simulink model "utolso"  (R2023b)
settings: Solver=FixedStepAuto  StartTime=0.0  StopTime=100  FixedStep=0.01  RelTol=1e-3
values from neighbouring files (symbols this model uses):
  A = [2 5 2.3; 1 0 3; 0 -4.1 5]    [elso_ora.m]    (also in laborXI.m = [0 1;-k/m -b/m])
  Ah = [A B; 0 0 0]    [laborXI.m]
  B = [1;-1;-2]    [elso_ora.m]    (also in laborXI.m = [0;1/m])
  Bh = [B;0]    [laborXI.m]
  C = [-1 -2 3]    [elso_ora.m]    (also in laborXI.m = [1 0])
  Ch = [C 0]    [laborXI.m]
  Gh = acker(Ah',Ch',[soh1 soh2 soh3])'    [laborXI.m]
  K = acker(A,B,[sc1 sc2])    [laborXI.m]
  Mu = Mxu(3)    [laborXI.m]
  Mx = Mxu(1:2)    [laborXI.m]
settings Model: Creator=andra  LastModifiedBy=andra

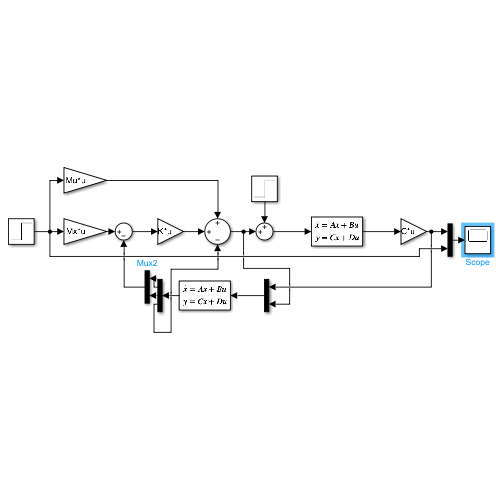
[thumbnail: Simulink's stored preview of the top-level diagram]
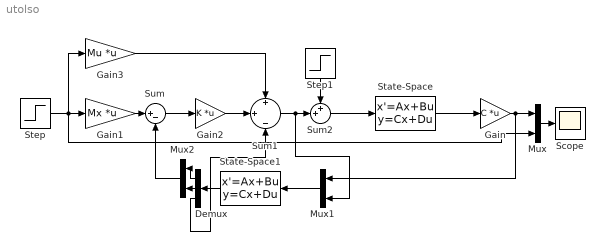
== system utolso ==
  Demux : Demux  Outputs=3
  Gain : Gain  Gain=C  Multiplication=Matrix(K*u)
  Gain1 : Gain  Gain=Mx  Multiplication=Matrix(K*u)
  Gain2 : Gain  Gain=K  Multiplication=Matrix(K*u)
  Gain3 : Gain  Gain=Mu  Multiplication=Matrix(K*u)
  Mux : Mux  Inputs=2
  Mux1 : Mux  Inputs=2
  Mux2 : Mux  Inputs=2
  Scope : Scope
  State-Space : StateSpace  A=A  B=B  C=eye(2)  D=zeros(2,1)  InitialCondition=[0.1 ; 0]
  State-Space1 : StateSpace  A=Ah-Gh*Ch  B=[Gh Bh]  C=eye(3)  D=zeros(3,2)  InitialCondition=0
  Step : Step  Time=40  SampleTime=0
  Step1 : Step  Time=70  After=10  SampleTime=0
  Sum : Sum  Inputs=|+-
  Sum1 : Sum  Inputs=+|+|-
  Sum2 : Sum  Inputs=++|
  wires:
  State-Space/1 -> Gain/1
  Gain/1 -> Mux/1, Mux1/1
  Mux/1 -> Scope/1
  Step/1 -> Mux/2, Gain1/1, Gain3/1
  Gain1/1 -> Sum/1
  Sum/1 -> Gain2/1
  Gain2/1 -> Sum1/2
  Gain3/1 -> Sum1/1
  Sum1/1 -> Sum2/2, Mux1/2
  Mux1/1 -> State-Space1/1
  State-Space1/1 -> Demux/1
  Demux/1 -> Mux2/1
  Demux/2 -> Mux2/2
  Mux2/1 -> Sum/2
  Demux/3 -> Sum1/3
  Sum2/1 -> State-Space/1
  Step1/1 -> Sum2/1
